simulink model "simRouteA_v4_11"  (R2015a)
settings: Solver=FixedStepDiscrete  StartTime=0.0  StopTime=36000  FixedStep=1  RelTol=1e-3
PreLoadFcn:
  | loadTimetable
StopFcn:
  | postProcess
undefined symbols (not defined in the file or in its folder): setBus1IntergenTime, setBus2IntergenTime, setBus3IntergenTime, setBus4IntergenTime
(part 6 of 7)

== system simRouteA_v4_11/chkSchedTimeNormalBusAtCP3/Subsystem2 ==
  ID : Inport
  tTable : Inport  Port=2
  Constant12 : Constant  Value=10000
  Constant13 : Constant
  Direct Lookup Table (n-D)1 : LookupNDDirect  TableIsInput=on
  Divide1 : Product  Inputs=/*
  Math Function1 : Math  Operator=mod  SaturateOnIntegerOverflow=on
  Rounding : Rounding  Operator=round
  Rounding1 : Rounding  Operator=round
  Subtract1 : Sum  Inputs=-+
  schedTime : Outport
  wires:
  Rounding1/1 -> Direct Lookup Table (n-D)1/1
  Constant12/1 -> Math Function1/2, Divide1/1
  Constant13/1 -> Subtract1/1
  Divide1/1 -> Rounding/1
  Subtract1/1 -> Direct Lookup Table (n-D)1/2
  Direct Lookup Table (n-D)1/1 -> schedTime/1
  tTable/1 -> Direct Lookup Table (n-D)1/3
  Math Function1/1 -> Rounding1/1
  Rounding/1 -> Subtract1/2
  ID/1 -> Divide1/2, Math Function1/1

== system simRouteA_v4_11/chkSchedTimeNormalBusAtCP3/While Iterator Subsystem ==
  crnBusID : Inport
  timetableAtStart : Inport  Port=2
  crnTimeAtCP : Inport  Port=3
  IC : Inport  Port=4
  Add1 : Sum
  Constant2 : Constant  Value=10000
  Constant4 : Constant
  Direct Lookup Table (n-D)2 : LookupNDDirect  TableIsInput=on
  Divide2 : Product  Inputs=/*
  Math Function1 : Math  Operator=mod  SaturateOnIntegerOverflow=on
  Memory : Memory
  Relational Operator : RelationalOperator  Operator=<=  OutDataTypeStr=boolean
  Rounding2 : Rounding  Operator=round
  Rounding3 : Rounding  Operator=round
  Subtract2 : Sum  Inputs=-+
  Sum : Sum  Inputs=|++
  While Iterator : WhileIterator  ShowIterationPort=on
  nxtDepTimeAtStart : Outport
  nxtBusID : Outport  Port=2
  wires:
  IC/1 -> While Iterator/2
  While Iterator/1 -> Sum/1
  Memory/1 -> Sum/2
  Sum/1 -> Add1/2, Memory/1
  crnBusID/1 -> Add1/1
  Rounding2/1 -> Direct Lookup Table (n-D)2/1
  Divide2/1 -> Rounding3/1
  Add1/1 -> Divide2/2, nxtBusID/1, Math Function1/1
  Math Function1/1 -> Rounding2/1
  Constant2/1 -> Divide2/1, Math Function1/2
  timetableAtStart/1 -> Direct Lookup Table (n-D)2/3
  Rounding3/1 -> Subtract2/2
  Constant4/1 -> Subtract2/1
  Subtract2/1 -> Direct Lookup Table (n-D)2/2
  Direct Lookup Table (n-D)2/1 -> Relational Operator/1, nxtDepTimeAtStart/1
  crnTimeAtCP/1 -> Relational Operator/2
  Relational Operator/1 -> While Iterator/1

== system simRouteA_v4_11/chkSchedTimeNormalBusAtCP4/Subsystem2 ==
  ID : Inport
  tTable : Inport  Port=2
  Constant12 : Constant  Value=10000
  Constant13 : Constant
  Direct Lookup Table (n-D)1 : LookupNDDirect  TableIsInput=on
  Divide1 : Product  Inputs=/*
  Math Function1 : Math  Operator=mod  SaturateOnIntegerOverflow=on
  Rounding : Rounding  Operator=round
  Rounding1 : Rounding  Operator=round
  Subtract1 : Sum  Inputs=-+
  schedTime : Outport
  wires:
  Rounding1/1 -> Direct Lookup Table (n-D)1/1
  Constant12/1 -> Math Function1/2, Divide1/1
  Constant13/1 -> Subtract1/1
  Divide1/1 -> Rounding/1
  Subtract1/1 -> Direct Lookup Table (n-D)1/2
  Direct Lookup Table (n-D)1/1 -> schedTime/1
  tTable/1 -> Direct Lookup Table (n-D)1/3
  Math Function1/1 -> Rounding1/1
  Rounding/1 -> Subtract1/2
  ID/1 -> Divide1/2, Math Function1/1

== system simRouteA_v4_11/chkSchedTimeNormalBusAtCP4/While Iterator Subsystem ==
  crnBusID : Inport
  timetableAtStart : Inport  Port=2
  crnTimeAtCP : Inport  Port=3
  IC : Inport  Port=4
  Add1 : Sum
  Constant2 : Constant  Value=10000
  Constant4 : Constant
  Direct Lookup Table (n-D)2 : LookupNDDirect  TableIsInput=on
  Divide2 : Product  Inputs=/*
  Math Function1 : Math  Operator=mod  SaturateOnIntegerOverflow=on
  Memory : Memory
  Relational Operator : RelationalOperator  Operator=<=  OutDataTypeStr=boolean
  Rounding2 : Rounding  Operator=round
  Rounding3 : Rounding  Operator=round
  Subtract2 : Sum  Inputs=-+
  Sum : Sum  Inputs=|++
  While Iterator : WhileIterator  ShowIterationPort=on
  nxtDepTimeAtStart : Outport
  nxtBusID : Outport  Port=2
  wires:
  IC/1 -> While Iterator/2
  While Iterator/1 -> Sum/1
  Memory/1 -> Sum/2
  Sum/1 -> Add1/2, Memory/1
  crnBusID/1 -> Add1/1
  Rounding2/1 -> Direct Lookup Table (n-D)2/1
  Divide2/1 -> Rounding3/1
  Add1/1 -> Divide2/2, nxtBusID/1, Math Function1/1
  Math Function1/1 -> Rounding2/1
  Constant2/1 -> Divide2/1, Math Function1/2
  timetableAtStart/1 -> Direct Lookup Table (n-D)2/3
  Rounding3/1 -> Subtract2/2
  Constant4/1 -> Subtract2/1
  Subtract2/1 -> Direct Lookup Table (n-D)2/2
  Direct Lookup Table (n-D)2/1 -> Relational Operator/1, nxtDepTimeAtStart/1
  crnTimeAtCP/1 -> Relational Operator/2
  Relational Operator/1 -> While Iterator/1

== system simRouteA_v4_11/holdBusAtCP2/While Iterator Subsystem ==
  crnBusID : Inport
  timetableAtStart : Inport  Port=2
  crnTimeAtCP : Inport  Port=3
  IC : Inport  Port=4
  Add1 : Sum
  Constant2 : Constant  Value=10000
  Constant4 : Constant
  Direct Lookup Table (n-D)2 : LookupNDDirect  TableIsInput=on
  Divide2 : Product  Inputs=/*
  Math Function1 : Math  Operator=mod  SaturateOnIntegerOverflow=on
  Memory : Memory
  Relational Operator : RelationalOperator  Operator=<=  OutDataTypeStr=boolean
  Rounding2 : Rounding  Operator=round
  Rounding3 : Rounding  Operator=round
  Subtract2 : Sum  Inputs=-+
  Sum : Sum  Inputs=|++
  While Iterator : WhileIterator  ShowIterationPort=on
  nxtDepTimeAtStart : Outport
  nxtBusID : Outport  Port=2
  wires:
  IC/1 -> While Iterator/2
  While Iterator/1 -> Sum/1
  Memory/1 -> Sum/2
  Sum/1 -> Add1/2, Memory/1
  crnBusID/1 -> Add1/1
  Rounding2/1 -> Direct Lookup Table (n-D)2/1
  Divide2/1 -> Rounding3/1
  Add1/1 -> Divide2/2, nxtBusID/1, Math Function1/1
  Math Function1/1 -> Rounding2/1
  Constant2/1 -> Divide2/1, Math Function1/2
  timetableAtStart/1 -> Direct Lookup Table (n-D)2/3
  Rounding3/1 -> Subtract2/2
  Constant4/1 -> Subtract2/1
  Subtract2/1 -> Direct Lookup Table (n-D)2/2
  Direct Lookup Table (n-D)2/1 -> Relational Operator/1, nxtDepTimeAtStart/1
  crnTimeAtCP/1 -> Relational Operator/2
  Relational Operator/1 -> While Iterator/1

== system simRouteA_v4_11/holdBusAtCP2/calculateHoldTimeAtCP ==
  crnSchedAtCP : Inport
  time : Inport  Port=2
  Constant2 : Constant  Value=0
  MinMax : MinMax  Function=max  Inputs=2
  Subtract1 : Sum  Inputs=+-
  tHoldCrnBus : Outport
  wires:
  Subtract1/1 -> MinMax/1
  MinMax/1 -> tHoldCrnBus/1
  Constant2/1 -> MinMax/2
  time/1 -> Subtract1/2
  crnSchedAtCP/1 -> Subtract1/1

== system simRouteA_v4_11/holdBusAtCP3/While Iterator Subsystem ==
  crnBusID : Inport
  timetableAtStart : Inport  Port=2
  crnTimeAtCP : Inport  Port=3
  IC : Inport  Port=4
  Add1 : Sum
  Constant2 : Constant  Value=10000
  Constant4 : Constant
  Direct Lookup Table (n-D)2 : LookupNDDirect  TableIsInput=on
  Divide2 : Product  Inputs=/*
  Math Function1 : Math  Operator=mod  SaturateOnIntegerOverflow=on
  Memory : Memory
  Relational Operator : RelationalOperator  Operator=<=  OutDataTypeStr=boolean
  Rounding2 : Rounding  Operator=round
  Rounding3 : Rounding  Operator=round
  Subtract2 : Sum  Inputs=-+
  Sum : Sum  Inputs=|++
  While Iterator : WhileIterator  ShowIterationPort=on
  nxtDepTimeAtStart : Outport
  nxtBusID : Outport  Port=2
  wires:
  IC/1 -> While Iterator/2
  While Iterator/1 -> Sum/1
  Memory/1 -> Sum/2
  Sum/1 -> Add1/2, Memory/1
  crnBusID/1 -> Add1/1
  Rounding2/1 -> Direct Lookup Table (n-D)2/1
  Divide2/1 -> Rounding3/1
  Add1/1 -> Divide2/2, nxtBusID/1, Math Function1/1
  Math Function1/1 -> Rounding2/1
  Constant2/1 -> Divide2/1, Math Function1/2
  timetableAtStart/1 -> Direct Lookup Table (n-D)2/3
  Rounding3/1 -> Subtract2/2
  Constant4/1 -> Subtract2/1
  Subtract2/1 -> Direct Lookup Table (n-D)2/2
  Direct Lookup Table (n-D)2/1 -> Relational Operator/1, nxtDepTimeAtStart/1
  crnTimeAtCP/1 -> Relational Operator/2
  Relational Operator/1 -> While Iterator/1

== system simRouteA_v4_11/holdBusAtCP3/calculateHoldTimeAtCP ==
  crnSchedAtCP : Inport
  time : Inport  Port=2
  Constant2 : Constant  Value=0
  MinMax : MinMax  Function=max  Inputs=2
  Subtract1 : Sum  Inputs=+-
  tHoldCrnBus : Outport
  wires:
  Subtract1/1 -> MinMax/1
  MinMax/1 -> tHoldCrnBus/1
  Constant2/1 -> MinMax/2
  time/1 -> Subtract1/2
  crnSchedAtCP/1 -> Subtract1/1

== system simRouteA_v4_11/holdBusAtCP4/While Iterator Subsystem ==
  crnBusID : Inport
  timetableAtStart : Inport  Port=2
  crnTimeAtCP : Inport  Port=3
  IC : Inport  Port=4
  Add1 : Sum
  Constant2 : Constant  Value=10000
  Constant4 : Constant
  Direct Lookup Table (n-D)2 : LookupNDDirect  TableIsInput=on
  Divide2 : Product  Inputs=/*
  Math Function1 : Math  Operator=mod  SaturateOnIntegerOverflow=on
  Memory : Memory
  Relational Operator : RelationalOperator  Operator=<=  OutDataTypeStr=boolean
  Rounding2 : Rounding  Operator=round
  Rounding3 : Rounding  Operator=round
  Subtract2 : Sum  Inputs=-+
  Sum : Sum  Inputs=|++
  While Iterator : WhileIterator  ShowIterationPort=on
  nxtDepTimeAtStart : Outport
  nxtBusID : Outport  Port=2
  wires:
  IC/1 -> While Iterator/2
  While Iterator/1 -> Sum/1
  Memory/1 -> Sum/2
  Sum/1 -> Add1/2, Memory/1
  crnBusID/1 -> Add1/1
  Rounding2/1 -> Direct Lookup Table (n-D)2/1
  Divide2/1 -> Rounding3/1
  Add1/1 -> Divide2/2, nxtBusID/1, Math Function1/1
  Math Function1/1 -> Rounding2/1
  Constant2/1 -> Divide2/1, Math Function1/2
  timetableAtStart/1 -> Direct Lookup Table (n-D)2/3
  Rounding3/1 -> Subtract2/2
  Constant4/1 -> Subtract2/1
  Subtract2/1 -> Direct Lookup Table (n-D)2/2
  Direct Lookup Table (n-D)2/1 -> Relational Operator/1, nxtDepTimeAtStart/1
  crnTimeAtCP/1 -> Relational Operator/2
  Relational Operator/1 -> While Iterator/1

== system simRouteA_v4_11/holdBusAtCP4/calculateHoldTimeAtCP ==
  crnSchedAtCP : Inport
  time : Inport  Port=2
  Constant2 : Constant  Value=0
  MinMax : MinMax  Function=max  Inputs=2
  Subtract1 : Sum  Inputs=+-
  tHoldCrnBus : Outport
  wires:
  Subtract1/1 -> MinMax/1
  MinMax/1 -> tHoldCrnBus/1
  Constant2/1 -> MinMax/2
  time/1 -> Subtract1/2
  crnSchedAtCP/1 -> Subtract1/1

== system simRouteA_v4_11/inTransitLinkL1/Subsystem2 ==
  tTrav : Inport
  tDep : Inport  Port=2
  Add1 : Sum
  Add2 : Sum
  Subtract : Sum  Inputs=+-
  Subtract1 : Sum  Inputs=+-
  Switch : Switch  Criteria=u2 > Threshold
  Unit Delay : UnitDelay  SampleTime=-1
  headWay : Constant  Value=3
  tTravNew : Outport
  wires:
  Subtract/1 -> Switch/2
  Switch/1 -> Subtract1/1, Unit Delay/1
  headWay/1 -> Add2/1
  tDep/1 -> Subtract1/2, Add1/2
  Add2/1 -> Switch/3
  tTrav/1 -> Add1/1
  Subtract1/1 -> tTravNew/1
  Add1/1 -> Switch/1, Subtract/1
  Unit Delay/1 -> Add2/2, Subtract/2

== system simRouteA_v4_11/inTransitLinkL10/Subsystem2 ==
  tTrav : Inport
  tDep : Inport  Port=2
  Add1 : Sum
  Add2 : Sum
  Subtract : Sum  Inputs=+-
  Subtract1 : Sum  Inputs=+-
  Switch : Switch  Criteria=u2 > Threshold
  Unit Delay : UnitDelay  SampleTime=-1
  headWay : Constant  Value=3
  tTravNew : Outport
  wires:
  Subtract/1 -> Switch/2
  Switch/1 -> Subtract1/1, Unit Delay/1
  headWay/1 -> Add2/1
  tDep/1 -> Subtract1/2, Add1/2
  Add2/1 -> Switch/3
  tTrav/1 -> Add1/1
  Subtract1/1 -> tTravNew/1
  Add1/1 -> Switch/1, Subtract/1
  Unit Delay/1 -> Add2/2, Subtract/2

== system simRouteA_v4_11/inTransitLinkL11/Subsystem2 ==
  tTrav : Inport
  tDep : Inport  Port=2
  Add1 : Sum
  Add2 : Sum
  Subtract : Sum  Inputs=+-
  Subtract1 : Sum  Inputs=+-
  Switch : Switch  Criteria=u2 > Threshold
  Unit Delay : UnitDelay  SampleTime=-1
  headWay : Constant  Value=3
  tTravNew : Outport
  wires:
  Subtract/1 -> Switch/2
  Switch/1 -> Subtract1/1, Unit Delay/1
  headWay/1 -> Add2/1
  tDep/1 -> Subtract1/2, Add1/2
  Add2/1 -> Switch/3
  tTrav/1 -> Add1/1
  Subtract1/1 -> tTravNew/1
  Add1/1 -> Switch/1, Subtract/1
  Unit Delay/1 -> Add2/2, Subtract/2

== system simRouteA_v4_11/inTransitLinkL12/Subsystem2 ==
  tTrav : Inport
  tDep : Inport  Port=2
  Add1 : Sum
  Add2 : Sum
  Subtract : Sum  Inputs=+-
  Subtract1 : Sum  Inputs=+-
  Switch : Switch  Criteria=u2 > Threshold
  Unit Delay : UnitDelay  SampleTime=-1
  headWay : Constant  Value=3
  tTravNew : Outport
  wires:
  Subtract/1 -> Switch/2
  Switch/1 -> Subtract1/1, Unit Delay/1
  headWay/1 -> Add2/1
  tDep/1 -> Subtract1/2, Add1/2
  Add2/1 -> Switch/3
  tTrav/1 -> Add1/1
  Subtract1/1 -> tTravNew/1
  Add1/1 -> Switch/1, Subtract/1
  Unit Delay/1 -> Add2/2, Subtract/2

== system simRouteA_v4_11/inTransitLinkL13/Subsystem2 ==
  tTrav : Inport
  tDep : Inport  Port=2
  Add1 : Sum
  Add2 : Sum
  Subtract : Sum  Inputs=+-
  Subtract1 : Sum  Inputs=+-
  Switch : Switch  Criteria=u2 > Threshold
  Unit Delay : UnitDelay  SampleTime=-1
  headWay : Constant  Value=3
  tTravNew : Outport
  wires:
  Subtract/1 -> Switch/2
  Switch/1 -> Subtract1/1, Unit Delay/1
  headWay/1 -> Add2/1
  tDep/1 -> Subtract1/2, Add1/2
  Add2/1 -> Switch/3
  tTrav/1 -> Add1/1
  Subtract1/1 -> tTravNew/1
  Add1/1 -> Switch/1, Subtract/1
  Unit Delay/1 -> Add2/2, Subtract/2

== system simRouteA_v4_11/inTransitLinkL14/Subsystem2 ==
  tTrav : Inport
  tDep : Inport  Port=2
  Add1 : Sum
  Add2 : Sum
  Subtract : Sum  Inputs=+-
  Subtract1 : Sum  Inputs=+-
  Switch : Switch  Criteria=u2 > Threshold
  Unit Delay : UnitDelay  SampleTime=-1
  headWay : Constant  Value=3
  tTravNew : Outport
  wires:
  Subtract/1 -> Switch/2
  Switch/1 -> Subtract1/1, Unit Delay/1
  headWay/1 -> Add2/1
  tDep/1 -> Subtract1/2, Add1/2
  Add2/1 -> Switch/3
  tTrav/1 -> Add1/1
  Subtract1/1 -> tTravNew/1
  Add1/1 -> Switch/1, Subtract/1
  Unit Delay/1 -> Add2/2, Subtract/2

== system simRouteA_v4_11/inTransitLinkL15/Subsystem2 ==
  tTrav : Inport
  tDep : Inport  Port=2
  Add1 : Sum
  Add2 : Sum
  Subtract : Sum  Inputs=+-
  Subtract1 : Sum  Inputs=+-
  Switch : Switch  Criteria=u2 > Threshold
  Unit Delay : UnitDelay  SampleTime=-1
  headWay : Constant  Value=3
  tTravNew : Outport
  wires:
  Subtract/1 -> Switch/2
  Switch/1 -> Subtract1/1, Unit Delay/1
  headWay/1 -> Add2/1
  tDep/1 -> Subtract1/2, Add1/2
  Add2/1 -> Switch/3
  tTrav/1 -> Add1/1
  Subtract1/1 -> tTravNew/1
  Add1/1 -> Switch/1, Subtract/1
  Unit Delay/1 -> Add2/2, Subtract/2

== system simRouteA_v4_11/inTransitLinkL16/Subsystem2 ==
  tTrav : Inport
  tDep : Inport  Port=2
  Add1 : Sum
  Add2 : Sum
  Subtract : Sum  Inputs=+-
  Subtract1 : Sum  Inputs=+-
  Switch : Switch  Criteria=u2 > Threshold
  Unit Delay : UnitDelay  SampleTime=-1
  headWay : Constant  Value=3
  tTravNew : Outport
  wires:
  Subtract/1 -> Switch/2
  Switch/1 -> Subtract1/1, Unit Delay/1
  headWay/1 -> Add2/1
  tDep/1 -> Subtract1/2, Add1/2
  Add2/1 -> Switch/3
  tTrav/1 -> Add1/1
  Subtract1/1 -> tTravNew/1
  Add1/1 -> Switch/1, Subtract/1
  Unit Delay/1 -> Add2/2, Subtract/2

== system simRouteA_v4_11/inTransitLinkL17/Subsystem2 ==
  tTrav : Inport
  tDep : Inport  Port=2
  Add1 : Sum
  Add2 : Sum
  Subtract : Sum  Inputs=+-
  Subtract1 : Sum  Inputs=+-
  Switch : Switch  Criteria=u2 > Threshold
  Unit Delay : UnitDelay  SampleTime=-1
  headWay : Constant  Value=3
  tTravNew : Outport
  wires:
  Subtract/1 -> Switch/2
  Switch/1 -> Subtract1/1, Unit Delay/1
  headWay/1 -> Add2/1
  tDep/1 -> Subtract1/2, Add1/2
  Add2/1 -> Switch/3
  tTrav/1 -> Add1/1
  Subtract1/1 -> tTravNew/1
  Add1/1 -> Switch/1, Subtract/1
  Unit Delay/1 -> Add2/2, Subtract/2

== system simRouteA_v4_11/inTransitLinkL18/Subsystem2 ==
  tTrav : Inport
  tDep : Inport  Port=2
  Add1 : Sum
  Add2 : Sum
  Subtract : Sum  Inputs=+-
  Subtract1 : Sum  Inputs=+-
  Switch : Switch  Criteria=u2 > Threshold
  Unit Delay : UnitDelay  SampleTime=-1
  headWay : Constant  Value=3
  tTravNew : Outport
  wires:
  Subtract/1 -> Switch/2
  Switch/1 -> Subtract1/1, Unit Delay/1
  headWay/1 -> Add2/1
  tDep/1 -> Subtract1/2, Add1/2
  Add2/1 -> Switch/3
  tTrav/1 -> Add1/1
  Subtract1/1 -> tTravNew/1
  Add1/1 -> Switch/1, Subtract/1
  Unit Delay/1 -> Add2/2, Subtract/2

== system simRouteA_v4_11/inTransitLinkL2/Subsystem2 ==
  tTrav : Inport
  tDep : Inport  Port=2
  Add1 : Sum
  Add2 : Sum
  Subtract : Sum  Inputs=+-
  Subtract1 : Sum  Inputs=+-
  Switch : Switch  Criteria=u2 > Threshold
  Unit Delay : UnitDelay  SampleTime=-1
  headWay : Constant  Value=3
  tTravNew : Outport
  wires:
  Subtract/1 -> Switch/2
  Switch/1 -> Subtract1/1, Unit Delay/1
  headWay/1 -> Add2/1
  tDep/1 -> Subtract1/2, Add1/2
  Add2/1 -> Switch/3
  tTrav/1 -> Add1/1
  Subtract1/1 -> tTravNew/1
  Add1/1 -> Switch/1, Subtract/1
  Unit Delay/1 -> Add2/2, Subtract/2

== system simRouteA_v4_11/inTransitLinkL3/Subsystem2 ==
  tTrav : Inport
  tDep : Inport  Port=2
  Add1 : Sum
  Add2 : Sum
  Subtract : Sum  Inputs=+-
  Subtract1 : Sum  Inputs=+-
  Switch : Switch  Criteria=u2 > Threshold
  Unit Delay : UnitDelay  SampleTime=-1
  headWay : Constant  Value=3
  tTravNew : Outport
  wires:
  Subtract/1 -> Switch/2
  Switch/1 -> Subtract1/1, Unit Delay/1
  headWay/1 -> Add2/1
  tDep/1 -> Subtract1/2, Add1/2
  Add2/1 -> Switch/3
  tTrav/1 -> Add1/1
  Subtract1/1 -> tTravNew/1
  Add1/1 -> Switch/1, Subtract/1
  Unit Delay/1 -> Add2/2, Subtract/2

== system simRouteA_v4_11/inTransitLinkL4/Subsystem2 ==
  tTrav : Inport
  tDep : Inport  Port=2
  Add1 : Sum
  Add2 : Sum
  Subtract : Sum  Inputs=+-
  Subtract1 : Sum  Inputs=+-
  Switch : Switch  Criteria=u2 > Threshold
  Unit Delay : UnitDelay  SampleTime=-1
  headWay : Constant  Value=3
  tTravNew : Outport
  wires:
  Subtract/1 -> Switch/2
  Switch/1 -> Subtract1/1, Unit Delay/1
  headWay/1 -> Add2/1
  tDep/1 -> Subtract1/2, Add1/2
  Add2/1 -> Switch/3
  tTrav/1 -> Add1/1
  Subtract1/1 -> tTravNew/1
  Add1/1 -> Switch/1, Subtract/1
  Unit Delay/1 -> Add2/2, Subtract/2

== system simRouteA_v4_11/inTransitLinkL5/Subsystem2 ==
  tTrav : Inport
  tDep : Inport  Port=2
  Add1 : Sum
  Add2 : Sum
  Subtract : Sum  Inputs=+-
  Subtract1 : Sum  Inputs=+-
  Switch : Switch  Criteria=u2 > Threshold
  Unit Delay : UnitDelay  SampleTime=-1
  headWay : Constant  Value=3
  tTravNew : Outport
  wires:
  Subtract/1 -> Switch/2
  Switch/1 -> Subtract1/1, Unit Delay/1
  headWay/1 -> Add2/1
  tDep/1 -> Subtract1/2, Add1/2
  Add2/1 -> Switch/3
  tTrav/1 -> Add1/1
  Subtract1/1 -> tTravNew/1
  Add1/1 -> Switch/1, Subtract/1
  Unit Delay/1 -> Add2/2, Subtract/2

== system simRouteA_v4_11/inTransitLinkL6/Subsystem2 ==
  tTrav : Inport
  tDep : Inport  Port=2
  Add1 : Sum
  Add2 : Sum
  Subtract : Sum  Inputs=+-
  Subtract1 : Sum  Inputs=+-
  Switch : Switch  Criteria=u2 > Threshold
  Unit Delay : UnitDelay  SampleTime=-1
  headWay : Constant  Value=3
  tTravNew : Outport
  wires:
  Subtract/1 -> Switch/2
  Switch/1 -> Subtract1/1, Unit Delay/1
  headWay/1 -> Add2/1
  tDep/1 -> Subtract1/2, Add1/2
  Add2/1 -> Switch/3
  tTrav/1 -> Add1/1
  Subtract1/1 -> tTravNew/1
  Add1/1 -> Switch/1, Subtract/1
  Unit Delay/1 -> Add2/2, Subtract/2

== system simRouteA_v4_11/inTransitLinkL7/Subsystem2 ==
  tTrav : Inport
  tDep : Inport  Port=2
  Add1 : Sum
  Add2 : Sum
  Subtract : Sum  Inputs=+-
  Subtract1 : Sum  Inputs=+-
  Switch : Switch  Criteria=u2 > Threshold
  Unit Delay : UnitDelay  SampleTime=-1
  headWay : Constant  Value=3
  tTravNew : Outport
  wires:
  Subtract/1 -> Switch/2
  Switch/1 -> Subtract1/1, Unit Delay/1
  headWay/1 -> Add2/1
  tDep/1 -> Subtract1/2, Add1/2
  Add2/1 -> Switch/3
  tTrav/1 -> Add1/1
  Subtract1/1 -> tTravNew/1
  Add1/1 -> Switch/1, Subtract/1
  Unit Delay/1 -> Add2/2, Subtract/2

== system simRouteA_v4_11/inTransitLinkL8/Subsystem2 ==
  tTrav : Inport
  tDep : Inport  Port=2
  Add1 : Sum
  Add2 : Sum
  Subtract : Sum  Inputs=+-
  Subtract1 : Sum  Inputs=+-
  Switch : Switch  Criteria=u2 > Threshold
  Unit Delay : UnitDelay  SampleTime=-1
  headWay : Constant  Value=3
  tTravNew : Outport
  wires:
  Subtract/1 -> Switch/2
  Switch/1 -> Subtract1/1, Unit Delay/1
  headWay/1 -> Add2/1
  tDep/1 -> Subtract1/2, Add1/2
  Add2/1 -> Switch/3
  tTrav/1 -> Add1/1
  Subtract1/1 -> tTravNew/1
  Add1/1 -> Switch/1, Subtract/1
  Unit Delay/1 -> Add2/2, Subtract/2

== system simRouteA_v4_11/inTransitLinkL9/Subsystem2 ==
  tTrav : Inport
  tDep : Inport  Port=2
  Add1 : Sum
  Add2 : Sum
  Subtract : Sum  Inputs=+-
  Subtract1 : Sum  Inputs=+-
  Switch : Switch  Criteria=u2 > Threshold
  Unit Delay : UnitDelay  SampleTime=-1
  headWay : Constant  Value=3
  tTravNew : Outport
  wires:
  Subtract/1 -> Switch/2
  Switch/1 -> Subtract1/1, Unit Delay/1
  headWay/1 -> Add2/1
  tDep/1 -> Subtract1/2, Add1/2
  Add2/1 -> Switch/3
  tTrav/1 -> Add1/1
  Subtract1/1 -> tTravNew/1
  Add1/1 -> Switch/1, Subtract/1
  Unit Delay/1 -> Add2/2, Subtract/2

== system simRouteA_v4_11/atStopS1/busDwellThisStop/Subsystem2 ==
  dwellTime : Inport
  tStartSrvPax : Inport  Port=2
  Add1 : Sum
  Add2 : Sum
  Subtract : Sum  Inputs=+-
  Subtract1 : Sum  Inputs=+-
  Switch : Switch  Criteria=u2 > Threshold
  Unit Delay : UnitDelay  SampleTime=-1
  headWay : Constant  Value=3
  dwellTimeNew : Outport
  wires:
  Subtract/1 -> Switch/2
  Switch/1 -> Subtract1/1, Unit Delay/1
  headWay/1 -> Add2/1
  tStartSrvPax/1 -> Subtract1/2, Add1/2
  Add2/1 -> Switch/3
  dwellTime/1 -> Add1/1
  Subtract1/1 -> dwellTimeNew/1
  Add1/1 -> Switch/1, Subtract/1
  Unit Delay/1 -> Add2/2, Subtract/2

== system simRouteA_v4_11/atStopS1/calcPaxActivThisStop/Atomic Subsystem ==
  maxCap : Inport
  vacancy : Inport  Port=2
  paxAlight : Inport  Port=3
  paxArr : Inport  Port=4
  sec2Brd : Inport  Port=5
  Add : Sum
  Add1 : Sum
  Add2 : Sum
  Initial Value : InitialValue  Commented=on  InitialValue=0
  Min1 : MinMax  Inputs=2
  Min2 : MinMax  Inputs=2
  Product : Product
  Signal Latch : SignalLatch  Commented=on  MemoryWriteEdgeOption=Either  MemoryReadEdgeOption=Either  SpecifyReadEventPriority=on
      settings: InputPortMap=u0,u1,u2  OutputPortMap=o2
  Subtract : Sum  Inputs=+-
  Subtract1 : Sum  Inputs=-+
  Subtract2 : Sum  Inputs=+-
  Unit Delay : UnitDelay  SampleTime=-1
  newVacancy : Outport
  paxBoard : Outport  Port=2
  paxRemain : Outport  Port=3
  paxWait : Outport  Port=4
  dwellTime : Outport  Port=5
  corrPaxAlight : Outport  Port=6
  wires:
  Add/1 -> Min1/1, Subtract/1
  Min1/1 -> Subtract1/1, Subtract/2, Add2/1, paxBoard/1
  paxArr/1 -> Add1/1
  Add1/1 -> paxWait/1, Subtract1/2, Min1/2
  Subtract1/1 -> Unit Delay/1, paxRemain/1
  Unit Delay/1 -> Add1/2
  vacancy/1 -> Subtract2/2, Add/1
  maxCap/1 -> Subtract2/1
  Subtract/1 -> newVacancy/1
  Add2/1 -> Product/1
  sec2Brd/1 -> Product/2
  Product/1 -> dwellTime/1
  Subtract2/1 -> Min2/1
  Min2/1 -> corrPaxAlight/1, Add2/2, Add/2
  paxAlight/1 -> Min2/2

== system simRouteA_v4_11/atStopS1/calcPaxActivThisStop/calcPaxAlightS1 ==
  integrPax : Inport
  Subtract : Sum  Inputs=+-
  Unit Delay : UnitDelay  SampleTime=-1
  truPax : Outport
  intgPax : Outport  Port=2
  wires:
  integrPax/1 -> Unit Delay/1, intgPax/1, Subtract/1
  Subtract/1 -> truPax/1
  Unit Delay/1 -> Subtract/2

== system simRouteA_v4_11/atStopS1/calcPaxActivThisStop/calcPaxArrS1 ==
  integrPax : Inport
  Subtract : Sum  Inputs=+-
  Unit Delay : UnitDelay  SampleTime=-1
  truPax : Outport
  intgPax : Outport  Port=2
  wires:
  integrPax/1 -> Unit Delay/1, intgPax/1, Subtract/1
  Subtract/1 -> truPax/1
  Unit Delay/1 -> Subtract/2

== system simRouteA_v4_11/atStopS1/integrPaxAlightS1/Atomic Subsystem1 ==
  In1 : Inport
  Add : Sum
  Unit Delay : UnitDelay  SampleTime=-1
  Out1 : Outport
  wires:
  In1/1 -> Add/1
  Add/1 -> Out1/1, Unit Delay/1
  Unit Delay/1 -> Add/2

== system simRouteA_v4_11/atStopS1/integrPaxArrS1/Atomic Subsystem1 ==
  In1 : Inport
  Add : Sum
  Unit Delay : UnitDelay  SampleTime=-1
  Out1 : Outport
  wires:
  In1/1 -> Add/1
  Add/1 -> Out1/1, Unit Delay/1
  Unit Delay/1 -> Add/2

== system simRouteA_v4_11/atStopS10/busDwellThisStop/Subsystem2 ==
  dwellTime : Inport
  tStartSrvPax : Inport  Port=2
  Add1 : Sum
  Add2 : Sum
  Subtract : Sum  Inputs=+-
  Subtract1 : Sum  Inputs=+-
  Switch : Switch  Criteria=u2 > Threshold
  Unit Delay : UnitDelay  SampleTime=-1
  headWay : Constant  Value=3
  dwellTimeNew : Outport
  wires:
  Subtract/1 -> Switch/2
  Switch/1 -> Subtract1/1, Unit Delay/1
  headWay/1 -> Add2/1
  tStartSrvPax/1 -> Subtract1/2, Add1/2
  Add2/1 -> Switch/3
  dwellTime/1 -> Add1/1
  Subtract1/1 -> dwellTimeNew/1
  Add1/1 -> Switch/1, Subtract/1
  Unit Delay/1 -> Add2/2, Subtract/2

== system simRouteA_v4_11/atStopS10/calcPaxActivThisStop/Atomic Subsystem ==
  maxCap : Inport
  vacancy : Inport  Port=2
  paxAlight : Inport  Port=3
  paxArr : Inport  Port=4
  sec2Brd : Inport  Port=5
  Add : Sum
  Add1 : Sum
  Add2 : Sum
  Initial Value : InitialValue  Commented=on  InitialValue=0
  Min1 : MinMax  Inputs=2
  Min2 : MinMax  Inputs=2
  Product : Product
  Signal Latch : SignalLatch  Commented=on  MemoryWriteEdgeOption=Either  MemoryReadEdgeOption=Either  SpecifyReadEventPriority=on
      settings: InputPortMap=u0,u1,u2  OutputPortMap=o2
  Subtract : Sum  Inputs=+-
  Subtract1 : Sum  Inputs=-+
  Subtract2 : Sum  Inputs=+-
  Unit Delay : UnitDelay  SampleTime=-1
  newVacancy : Outport
  paxBoard : Outport  Port=2
  paxRemain : Outport  Port=3
  paxWait : Outport  Port=4
  dwellTime : Outport  Port=5
  corrPaxAlight : Outport  Port=6
  wires:
  Add/1 -> Min1/1, Subtract/1
  Min1/1 -> Subtract1/1, Subtract/2, Add2/1, paxBoard/1
  paxArr/1 -> Add1/1
  Add1/1 -> paxWait/1, Subtract1/2, Min1/2
  Subtract1/1 -> Unit Delay/1, paxRemain/1
  Unit Delay/1 -> Add1/2
  vacancy/1 -> Subtract2/2, Add/1
  maxCap/1 -> Subtract2/1
  Subtract/1 -> newVacancy/1
  Add2/1 -> Product/1
  sec2Brd/1 -> Product/2
  Product/1 -> dwellTime/1
  Subtract2/1 -> Min2/1
  Min2/1 -> corrPaxAlight/1, Add2/2, Add/2
  paxAlight/1 -> Min2/2

== system simRouteA_v4_11/atStopS10/calcPaxActivThisStop/calcPaxAlightS1 ==
  integrPax : Inport
  Subtract : Sum  Inputs=+-
  Unit Delay : UnitDelay  SampleTime=-1
  truPax : Outport
  intgPax : Outport  Port=2
  wires:
  integrPax/1 -> Unit Delay/1, intgPax/1, Subtract/1
  Subtract/1 -> truPax/1
  Unit Delay/1 -> Subtract/2

== system simRouteA_v4_11/atStopS10/calcPaxActivThisStop/calcPaxArrS1 ==
  integrPax : Inport
  Subtract : Sum  Inputs=+-
  Unit Delay : UnitDelay  SampleTime=-1
  truPax : Outport
  intgPax : Outport  Port=2
  wires:
  integrPax/1 -> Unit Delay/1, intgPax/1, Subtract/1
  Subtract/1 -> truPax/1
  Unit Delay/1 -> Subtract/2

== system simRouteA_v4_11/atStopS10/integrPaxAlightS1/Atomic Subsystem1 ==
  In1 : Inport
  Add : Sum
  Unit Delay : UnitDelay  SampleTime=-1
  Out1 : Outport
  wires:
  In1/1 -> Add/1
  Add/1 -> Out1/1, Unit Delay/1
  Unit Delay/1 -> Add/2

== system simRouteA_v4_11/atStopS10/integrPaxArrS1/Atomic Subsystem1 ==
  In1 : Inport
  Add : Sum
  Unit Delay : UnitDelay  SampleTime=-1
  Out1 : Outport
  wires:
  In1/1 -> Add/1
  Add/1 -> Out1/1, Unit Delay/1
  Unit Delay/1 -> Add/2

== system simRouteA_v4_11/atStopS11/busDwellThisStop/Subsystem2 ==
  dwellTime : Inport
  tStartSrvPax : Inport  Port=2
  Add1 : Sum
  Add2 : Sum
  Subtract : Sum  Inputs=+-
  Subtract1 : Sum  Inputs=+-
  Switch : Switch  Criteria=u2 > Threshold
  Unit Delay : UnitDelay  SampleTime=-1
  headWay : Constant  Value=3
  dwellTimeNew : Outport
  wires:
  Subtract/1 -> Switch/2
  Switch/1 -> Subtract1/1, Unit Delay/1
  headWay/1 -> Add2/1
  tStartSrvPax/1 -> Subtract1/2, Add1/2
  Add2/1 -> Switch/3
  dwellTime/1 -> Add1/1
  Subtract1/1 -> dwellTimeNew/1
  Add1/1 -> Switch/1, Subtract/1
  Unit Delay/1 -> Add2/2, Subtract/2

== system simRouteA_v4_11/atStopS11/calcPaxActivThisStop/Atomic Subsystem ==
  maxCap : Inport
  vacancy : Inport  Port=2
  paxAlight : Inport  Port=3
  paxArr : Inport  Port=4
  sec2Brd : Inport  Port=5
  Add : Sum
  Add1 : Sum
  Add2 : Sum
  Initial Value : InitialValue  Commented=on  InitialValue=0
  Min1 : MinMax  Inputs=2
  Min2 : MinMax  Inputs=2
  Product : Product
  Signal Latch : SignalLatch  Commented=on  MemoryWriteEdgeOption=Either  MemoryReadEdgeOption=Either  SpecifyReadEventPriority=on
      settings: InputPortMap=u0,u1,u2  OutputPortMap=o2
  Subtract : Sum  Inputs=+-
  Subtract1 : Sum  Inputs=-+
  Subtract2 : Sum  Inputs=+-
  Unit Delay : UnitDelay  SampleTime=-1
  newVacancy : Outport
  paxBoard : Outport  Port=2
  paxRemain : Outport  Port=3
  paxWait : Outport  Port=4
  dwellTime : Outport  Port=5
  corrPaxAlight : Outport  Port=6
  wires:
  Add/1 -> Min1/1, Subtract/1
  Min1/1 -> Subtract1/1, Subtract/2, Add2/1, paxBoard/1
  paxArr/1 -> Add1/1
  Add1/1 -> paxWait/1, Subtract1/2, Min1/2
  Subtract1/1 -> Unit Delay/1, paxRemain/1
  Unit Delay/1 -> Add1/2
  vacancy/1 -> Subtract2/2, Add/1
  maxCap/1 -> Subtract2/1
  Subtract/1 -> newVacancy/1
  Add2/1 -> Product/1
  sec2Brd/1 -> Product/2
  Product/1 -> dwellTime/1
  Subtract2/1 -> Min2/1
  Min2/1 -> corrPaxAlight/1, Add2/2, Add/2
  paxAlight/1 -> Min2/2

== system simRouteA_v4_11/atStopS11/calcPaxActivThisStop/calcPaxAlightS1 ==
  integrPax : Inport
  Subtract : Sum  Inputs=+-
  Unit Delay : UnitDelay  SampleTime=-1
  truPax : Outport
  intgPax : Outport  Port=2
  wires:
  integrPax/1 -> Unit Delay/1, intgPax/1, Subtract/1
  Subtract/1 -> truPax/1
  Unit Delay/1 -> Subtract/2

== system simRouteA_v4_11/atStopS11/calcPaxActivThisStop/calcPaxArrS1 ==
  integrPax : Inport
  Subtract : Sum  Inputs=+-
  Unit Delay : UnitDelay  SampleTime=-1
  truPax : Outport
  intgPax : Outport  Port=2
  wires:
  integrPax/1 -> Unit Delay/1, intgPax/1, Subtract/1
  Subtract/1 -> truPax/1
  Unit Delay/1 -> Subtract/2

== system simRouteA_v4_11/atStopS11/integrPaxAlightS1/Atomic Subsystem1 ==
  In1 : Inport
  Add : Sum
  Unit Delay : UnitDelay  SampleTime=-1
  Out1 : Outport
  wires:
  In1/1 -> Add/1
  Add/1 -> Out1/1, Unit Delay/1
  Unit Delay/1 -> Add/2

== system simRouteA_v4_11/atStopS11/integrPaxArrS1/Atomic Subsystem1 ==
  In1 : Inport
  Add : Sum
  Unit Delay : UnitDelay  SampleTime=-1
  Out1 : Outport
  wires:
  In1/1 -> Add/1
  Add/1 -> Out1/1, Unit Delay/1
  Unit Delay/1 -> Add/2

== system simRouteA_v4_11/atStopS12/busDwellThisStop/Subsystem2 ==
  dwellTime : Inport
  tStartSrvPax : Inport  Port=2
  Add1 : Sum
  Add2 : Sum
  Subtract : Sum  Inputs=+-
  Subtract1 : Sum  Inputs=+-
  Switch : Switch  Criteria=u2 > Threshold
  Unit Delay : UnitDelay  SampleTime=-1
  headWay : Constant  Value=3
  dwellTimeNew : Outport
  wires:
  Subtract/1 -> Switch/2
  Switch/1 -> Subtract1/1, Unit Delay/1
  headWay/1 -> Add2/1
  tStartSrvPax/1 -> Subtract1/2, Add1/2
  Add2/1 -> Switch/3
  dwellTime/1 -> Add1/1
  Subtract1/1 -> dwellTimeNew/1
  Add1/1 -> Switch/1, Subtract/1
  Unit Delay/1 -> Add2/2, Subtract/2

== system simRouteA_v4_11/atStopS12/calcPaxActivThisStop/Atomic Subsystem ==
  maxCap : Inport
  vacancy : Inport  Port=2
  paxAlight : Inport  Port=3
  paxArr : Inport  Port=4
  sec2Brd : Inport  Port=5
  Add : Sum
  Add1 : Sum
  Add2 : Sum
  Initial Value : InitialValue  Commented=on  InitialValue=0
  Min1 : MinMax  Inputs=2
  Min2 : MinMax  Inputs=2
  Product : Product
  Signal Latch : SignalLatch  Commented=on  MemoryWriteEdgeOption=Either  MemoryReadEdgeOption=Either  SpecifyReadEventPriority=on
      settings: InputPortMap=u0,u1,u2  OutputPortMap=o2
  Subtract : Sum  Inputs=+-
  Subtract1 : Sum  Inputs=-+
  Subtract2 : Sum  Inputs=+-
  Unit Delay : UnitDelay  SampleTime=-1
  newVacancy : Outport
  paxBoard : Outport  Port=2
  paxRemain : Outport  Port=3
  paxWait : Outport  Port=4
  dwellTime : Outport  Port=5
  corrPaxAlight : Outport  Port=6
  wires:
  Add/1 -> Min1/1, Subtract/1
  Min1/1 -> Subtract1/1, Subtract/2, Add2/1, paxBoard/1
  paxArr/1 -> Add1/1
  Add1/1 -> paxWait/1, Subtract1/2, Min1/2
  Subtract1/1 -> Unit Delay/1, paxRemain/1
  Unit Delay/1 -> Add1/2
  vacancy/1 -> Subtract2/2, Add/1
  maxCap/1 -> Subtract2/1
  Subtract/1 -> newVacancy/1
  Add2/1 -> Product/1
  sec2Brd/1 -> Product/2
  Product/1 -> dwellTime/1
  Subtract2/1 -> Min2/1
  Min2/1 -> corrPaxAlight/1, Add2/2, Add/2
  paxAlight/1 -> Min2/2

== system simRouteA_v4_11/atStopS12/calcPaxActivThisStop/calcPaxAlightS1 ==
  integrPax : Inport
  Subtract : Sum  Inputs=+-
  Unit Delay : UnitDelay  SampleTime=-1
  truPax : Outport
  intgPax : Outport  Port=2
  wires:
  integrPax/1 -> Unit Delay/1, intgPax/1, Subtract/1
  Subtract/1 -> truPax/1
  Unit Delay/1 -> Subtract/2

== system simRouteA_v4_11/atStopS12/calcPaxActivThisStop/calcPaxArrS1 ==
  integrPax : Inport
  Subtract : Sum  Inputs=+-
  Unit Delay : UnitDelay  SampleTime=-1
  truPax : Outport
  intgPax : Outport  Port=2
  wires:
  integrPax/1 -> Unit Delay/1, intgPax/1, Subtract/1
  Subtract/1 -> truPax/1
  Unit Delay/1 -> Subtract/2

== system simRouteA_v4_11/atStopS12/integrPaxAlightS1/Atomic Subsystem1 ==
  In1 : Inport
  Add : Sum
  Unit Delay : UnitDelay  SampleTime=-1
  Out1 : Outport
  wires:
  In1/1 -> Add/1
  Add/1 -> Out1/1, Unit Delay/1
  Unit Delay/1 -> Add/2

== system simRouteA_v4_11/atStopS12/integrPaxArrS1/Atomic Subsystem1 ==
  In1 : Inport
  Add : Sum
  Unit Delay : UnitDelay  SampleTime=-1
  Out1 : Outport
  wires:
  In1/1 -> Add/1
  Add/1 -> Out1/1, Unit Delay/1
  Unit Delay/1 -> Add/2

== system simRouteA_v4_11/atStopS13/busDwellThisStop/Subsystem2 ==
  dwellTime : Inport
  tStartSrvPax : Inport  Port=2
  Add1 : Sum
  Add2 : Sum
  Subtract : Sum  Inputs=+-
  Subtract1 : Sum  Inputs=+-
  Switch : Switch  Criteria=u2 > Threshold
  Unit Delay : UnitDelay  SampleTime=-1
  headWay : Constant  Value=3
  dwellTimeNew : Outport
  wires:
  Subtract/1 -> Switch/2
  Switch/1 -> Subtract1/1, Unit Delay/1
  headWay/1 -> Add2/1
  tStartSrvPax/1 -> Subtract1/2, Add1/2
  Add2/1 -> Switch/3
  dwellTime/1 -> Add1/1
  Subtract1/1 -> dwellTimeNew/1
  Add1/1 -> Switch/1, Subtract/1
  Unit Delay/1 -> Add2/2, Subtract/2

== system simRouteA_v4_11/atStopS13/calcPaxActivThisStop/Atomic Subsystem ==
  maxCap : Inport
  vacancy : Inport  Port=2
  paxAlight : Inport  Port=3
  paxArr : Inport  Port=4
  sec2Brd : Inport  Port=5
  Add : Sum
  Add1 : Sum
  Add2 : Sum
  Initial Value : InitialValue  Commented=on  InitialValue=0
  Min1 : MinMax  Inputs=2
  Min2 : MinMax  Inputs=2
  Product : Product
  Signal Latch : SignalLatch  Commented=on  MemoryWriteEdgeOption=Either  MemoryReadEdgeOption=Either  SpecifyReadEventPriority=on
      settings: InputPortMap=u0,u1,u2  OutputPortMap=o2
  Subtract : Sum  Inputs=+-
  Subtract1 : Sum  Inputs=-+
  Subtract2 : Sum  Inputs=+-
  Unit Delay : UnitDelay  SampleTime=-1
  newVacancy : Outport
  paxBoard : Outport  Port=2
  paxRemain : Outport  Port=3
  paxWait : Outport  Port=4
  dwellTime : Outport  Port=5
  corrPaxAlight : Outport  Port=6
  wires:
  Add/1 -> Min1/1, Subtract/1
  Min1/1 -> Subtract1/1, Subtract/2, Add2/1, paxBoard/1
  paxArr/1 -> Add1/1
  Add1/1 -> paxWait/1, Subtract1/2, Min1/2
  Subtract1/1 -> Unit Delay/1, paxRemain/1
  Unit Delay/1 -> Add1/2
  vacancy/1 -> Subtract2/2, Add/1
  maxCap/1 -> Subtract2/1
  Subtract/1 -> newVacancy/1
  Add2/1 -> Product/1
  sec2Brd/1 -> Product/2
  Product/1 -> dwellTime/1
  Subtract2/1 -> Min2/1
  Min2/1 -> corrPaxAlight/1, Add2/2, Add/2
  paxAlight/1 -> Min2/2

== system simRouteA_v4_11/atStopS13/calcPaxActivThisStop/calcPaxAlightS1 ==
  integrPax : Inport
  Subtract : Sum  Inputs=+-
  Unit Delay : UnitDelay  SampleTime=-1
  truPax : Outport
  intgPax : Outport  Port=2
  wires:
  integrPax/1 -> Unit Delay/1, intgPax/1, Subtract/1
  Subtract/1 -> truPax/1
  Unit Delay/1 -> Subtract/2

== system simRouteA_v4_11/atStopS13/calcPaxActivThisStop/calcPaxArrS1 ==
  integrPax : Inport
  Subtract : Sum  Inputs=+-
  Unit Delay : UnitDelay  SampleTime=-1
  truPax : Outport
  intgPax : Outport  Port=2
  wires:
  integrPax/1 -> Unit Delay/1, intgPax/1, Subtract/1
  Subtract/1 -> truPax/1
  Unit Delay/1 -> Subtract/2

== system simRouteA_v4_11/atStopS13/integrPaxAlightS1/Atomic Subsystem1 ==
  In1 : Inport
  Add : Sum
  Unit Delay : UnitDelay  SampleTime=-1
  Out1 : Outport
  wires:
  In1/1 -> Add/1
  Add/1 -> Out1/1, Unit Delay/1
  Unit Delay/1 -> Add/2

== system simRouteA_v4_11/atStopS13/integrPaxArrS1/Atomic Subsystem1 ==
  In1 : Inport
  Add : Sum
  Unit Delay : UnitDelay  SampleTime=-1
  Out1 : Outport
  wires:
  In1/1 -> Add/1
  Add/1 -> Out1/1, Unit Delay/1
  Unit Delay/1 -> Add/2

== system simRouteA_v4_11/atStopS14/busDwellThisStop/Subsystem2 ==
  dwellTime : Inport
  tStartSrvPax : Inport  Port=2
  Add1 : Sum
  Add2 : Sum
  Subtract : Sum  Inputs=+-
  Subtract1 : Sum  Inputs=+-
  Switch : Switch  Criteria=u2 > Threshold
  Unit Delay : UnitDelay  SampleTime=-1
  headWay : Constant  Value=3
  dwellTimeNew : Outport
  wires:
  Subtract/1 -> Switch/2
  Switch/1 -> Subtract1/1, Unit Delay/1
  headWay/1 -> Add2/1
  tStartSrvPax/1 -> Subtract1/2, Add1/2
  Add2/1 -> Switch/3
  dwellTime/1 -> Add1/1
  Subtract1/1 -> dwellTimeNew/1
  Add1/1 -> Switch/1, Subtract/1
  Unit Delay/1 -> Add2/2, Subtract/2

== system simRouteA_v4_11/atStopS14/calcPaxActivThisStop/Atomic Subsystem ==
  maxCap : Inport
  vacancy : Inport  Port=2
  paxAlight : Inport  Port=3
  paxArr : Inport  Port=4
  sec2Brd : Inport  Port=5
  Add : Sum
  Add1 : Sum
  Add2 : Sum
  Initial Value : InitialValue  Commented=on  InitialValue=0
  Min1 : MinMax  Inputs=2
  Min2 : MinMax  Inputs=2
  Product : Product
  Signal Latch : SignalLatch  Commented=on  MemoryWriteEdgeOption=Either  MemoryReadEdgeOption=Either  SpecifyReadEventPriority=on
      settings: InputPortMap=u0,u1,u2  OutputPortMap=o2
  Subtract : Sum  Inputs=+-
  Subtract1 : Sum  Inputs=-+
  Subtract2 : Sum  Inputs=+-
  Unit Delay : UnitDelay  SampleTime=-1
  newVacancy : Outport
  paxBoard : Outport  Port=2
  paxRemain : Outport  Port=3
  paxWait : Outport  Port=4
  dwellTime : Outport  Port=5
  corrPaxAlight : Outport  Port=6
  wires:
  Add/1 -> Min1/1, Subtract/1
  Min1/1 -> Subtract1/1, Subtract/2, Add2/1, paxBoard/1
  paxArr/1 -> Add1/1
  Add1/1 -> paxWait/1, Subtract1/2, Min1/2
  Subtract1/1 -> Unit Delay/1, paxRemain/1
  Unit Delay/1 -> Add1/2
  vacancy/1 -> Subtract2/2, Add/1
  maxCap/1 -> Subtract2/1
  Subtract/1 -> newVacancy/1
  Add2/1 -> Product/1
  sec2Brd/1 -> Product/2
  Product/1 -> dwellTime/1
  Subtract2/1 -> Min2/1
  Min2/1 -> corrPaxAlight/1, Add2/2, Add/2
  paxAlight/1 -> Min2/2

== system simRouteA_v4_11/atStopS14/calcPaxActivThisStop/calcPaxAlightS1 ==
  integrPax : Inport
  Subtract : Sum  Inputs=+-
  Unit Delay : UnitDelay  SampleTime=-1
  truPax : Outport
  intgPax : Outport  Port=2
  wires:
  integrPax/1 -> Unit Delay/1, intgPax/1, Subtract/1
  Subtract/1 -> truPax/1
  Unit Delay/1 -> Subtract/2

== system simRouteA_v4_11/atStopS14/calcPaxActivThisStop/calcPaxArrS1 ==
  integrPax : Inport
  Subtract : Sum  Inputs=+-
  Unit Delay : UnitDelay  SampleTime=-1
  truPax : Outport
  intgPax : Outport  Port=2
  wires:
  integrPax/1 -> Unit Delay/1, intgPax/1, Subtract/1
  Subtract/1 -> truPax/1
  Unit Delay/1 -> Subtract/2

== system simRouteA_v4_11/atStopS14/integrPaxAlightS1/Atomic Subsystem1 ==
  In1 : Inport
  Add : Sum
  Unit Delay : UnitDelay  SampleTime=-1
  Out1 : Outport
  wires:
  In1/1 -> Add/1
  Add/1 -> Out1/1, Unit Delay/1
  Unit Delay/1 -> Add/2

== system simRouteA_v4_11/atStopS14/integrPaxArrS1/Atomic Subsystem1 ==
  In1 : Inport
  Add : Sum
  Unit Delay : UnitDelay  SampleTime=-1
  Out1 : Outport
  wires:
  In1/1 -> Add/1
  Add/1 -> Out1/1, Unit Delay/1
  Unit Delay/1 -> Add/2

== system simRouteA_v4_11/atStopS15/busDwellThisStop/Subsystem2 ==
  dwellTime : Inport
  tStartSrvPax : Inport  Port=2
  Add1 : Sum
  Add2 : Sum
  Subtract : Sum  Inputs=+-
  Subtract1 : Sum  Inputs=+-
  Switch : Switch  Criteria=u2 > Threshold
  Unit Delay : UnitDelay  SampleTime=-1
  headWay : Constant  Value=3
  dwellTimeNew : Outport
  wires:
  Subtract/1 -> Switch/2
  Switch/1 -> Subtract1/1, Unit Delay/1
  headWay/1 -> Add2/1
  tStartSrvPax/1 -> Subtract1/2, Add1/2
  Add2/1 -> Switch/3
  dwellTime/1 -> Add1/1
  Subtract1/1 -> dwellTimeNew/1
  Add1/1 -> Switch/1, Subtract/1
  Unit Delay/1 -> Add2/2, Subtract/2

== system simRouteA_v4_11/atStopS15/calcPaxActivThisStop/Atomic Subsystem ==
  maxCap : Inport
  vacancy : Inport  Port=2
  paxAlight : Inport  Port=3
  paxArr : Inport  Port=4
  sec2Brd : Inport  Port=5
  Add : Sum
  Add1 : Sum
  Add2 : Sum
  Initial Value : InitialValue  Commented=on  InitialValue=0
  Min1 : MinMax  Inputs=2
  Min2 : MinMax  Inputs=2
  Product : Product
  Signal Latch : SignalLatch  Commented=on  MemoryWriteEdgeOption=Either  MemoryReadEdgeOption=Either  SpecifyReadEventPriority=on
      settings: InputPortMap=u0,u1,u2  OutputPortMap=o2
  Subtract : Sum  Inputs=+-
  Subtract1 : Sum  Inputs=-+
  Subtract2 : Sum  Inputs=+-
  Unit Delay : UnitDelay  SampleTime=-1
  newVacancy : Outport
  paxBoard : Outport  Port=2
  paxRemain : Outport  Port=3
  paxWait : Outport  Port=4
  dwellTime : Outport  Port=5
  corrPaxAlight : Outport  Port=6
  wires:
  Add/1 -> Min1/1, Subtract/1
  Min1/1 -> Subtract1/1, Subtract/2, Add2/1, paxBoard/1
  paxArr/1 -> Add1/1
  Add1/1 -> paxWait/1, Subtract1/2, Min1/2
  Subtract1/1 -> Unit Delay/1, paxRemain/1
  Unit Delay/1 -> Add1/2
  vacancy/1 -> Subtract2/2, Add/1
  maxCap/1 -> Subtract2/1
  Subtract/1 -> newVacancy/1
  Add2/1 -> Product/1
  sec2Brd/1 -> Product/2
  Product/1 -> dwellTime/1
  Subtract2/1 -> Min2/1
  Min2/1 -> corrPaxAlight/1, Add2/2, Add/2
  paxAlight/1 -> Min2/2

== system simRouteA_v4_11/atStopS15/calcPaxActivThisStop/calcPaxAlightS1 ==
  integrPax : Inport
  Subtract : Sum  Inputs=+-
  Unit Delay : UnitDelay  SampleTime=-1
  truPax : Outport
  intgPax : Outport  Port=2
  wires:
  integrPax/1 -> Unit Delay/1, intgPax/1, Subtract/1
  Subtract/1 -> truPax/1
  Unit Delay/1 -> Subtract/2

== system simRouteA_v4_11/atStopS15/calcPaxActivThisStop/calcPaxArrS1 ==
  integrPax : Inport
  Subtract : Sum  Inputs=+-
  Unit Delay : UnitDelay  SampleTime=-1
  truPax : Outport
  intgPax : Outport  Port=2
  wires:
  integrPax/1 -> Unit Delay/1, intgPax/1, Subtract/1
  Subtract/1 -> truPax/1
  Unit Delay/1 -> Subtract/2

== system simRouteA_v4_11/atStopS15/integrPaxAlightS1/Atomic Subsystem1 ==
  In1 : Inport
  Add : Sum
  Unit Delay : UnitDelay  SampleTime=-1
  Out1 : Outport
  wires:
  In1/1 -> Add/1
  Add/1 -> Out1/1, Unit Delay/1
  Unit Delay/1 -> Add/2

== system simRouteA_v4_11/atStopS15/integrPaxArrS1/Atomic Subsystem1 ==
  In1 : Inport
  Add : Sum
  Unit Delay : UnitDelay  SampleTime=-1
  Out1 : Outport
  wires:
  In1/1 -> Add/1
  Add/1 -> Out1/1, Unit Delay/1
  Unit Delay/1 -> Add/2

== system simRouteA_v4_11/atStopS16/busDwellThisStop/Subsystem2 ==
  dwellTime : Inport
  tStartSrvPax : Inport  Port=2
  Add1 : Sum
  Add2 : Sum
  Subtract : Sum  Inputs=+-
  Subtract1 : Sum  Inputs=+-
  Switch : Switch  Criteria=u2 > Threshold
  Unit Delay : UnitDelay  SampleTime=-1
  headWay : Constant  Value=3
  dwellTimeNew : Outport
  wires:
  Subtract/1 -> Switch/2
  Switch/1 -> Subtract1/1, Unit Delay/1
  headWay/1 -> Add2/1
  tStartSrvPax/1 -> Subtract1/2, Add1/2
  Add2/1 -> Switch/3
  dwellTime/1 -> Add1/1
  Subtract1/1 -> dwellTimeNew/1
  Add1/1 -> Switch/1, Subtract/1
  Unit Delay/1 -> Add2/2, Subtract/2

== system simRouteA_v4_11/atStopS16/calcPaxActivThisStop/Atomic Subsystem ==
  maxCap : Inport
  vacancy : Inport  Port=2
  paxAlight : Inport  Port=3
  paxArr : Inport  Port=4
  sec2Brd : Inport  Port=5
  Add : Sum
  Add1 : Sum
  Add2 : Sum
  Initial Value : InitialValue  Commented=on  InitialValue=0
  Min1 : MinMax  Inputs=2
  Min2 : MinMax  Inputs=2
  Product : Product
  Signal Latch : SignalLatch  Commented=on  MemoryWriteEdgeOption=Either  MemoryReadEdgeOption=Either  SpecifyReadEventPriority=on
      settings: InputPortMap=u0,u1,u2  OutputPortMap=o2
  Subtract : Sum  Inputs=+-
  Subtract1 : Sum  Inputs=-+
  Subtract2 : Sum  Inputs=+-
  Unit Delay : UnitDelay  SampleTime=-1
  newVacancy : Outport
  paxBoard : Outport  Port=2
  paxRemain : Outport  Port=3
  paxWait : Outport  Port=4
  dwellTime : Outport  Port=5
  corrPaxAlight : Outport  Port=6
  wires:
  Add/1 -> Min1/1, Subtract/1
  Min1/1 -> Subtract1/1, Subtract/2, Add2/1, paxBoard/1
  paxArr/1 -> Add1/1
  Add1/1 -> paxWait/1, Subtract1/2, Min1/2
  Subtract1/1 -> Unit Delay/1, paxRemain/1
  Unit Delay/1 -> Add1/2
  vacancy/1 -> Subtract2/2, Add/1
  maxCap/1 -> Subtract2/1
  Subtract/1 -> newVacancy/1
  Add2/1 -> Product/1
  sec2Brd/1 -> Product/2
  Product/1 -> dwellTime/1
  Subtract2/1 -> Min2/1
  Min2/1 -> corrPaxAlight/1, Add2/2, Add/2
  paxAlight/1 -> Min2/2

== system simRouteA_v4_11/atStopS16/calcPaxActivThisStop/calcPaxAlightS1 ==
  integrPax : Inport
  Subtract : Sum  Inputs=+-
  Unit Delay : UnitDelay  SampleTime=-1
  truPax : Outport
  intgPax : Outport  Port=2
  wires:
  integrPax/1 -> Unit Delay/1, intgPax/1, Subtract/1
  Subtract/1 -> truPax/1
  Unit Delay/1 -> Subtract/2

== system simRouteA_v4_11/atStopS16/calcPaxActivThisStop/calcPaxArrS1 ==
  integrPax : Inport
  Subtract : Sum  Inputs=+-
  Unit Delay : UnitDelay  SampleTime=-1
  truPax : Outport
  intgPax : Outport  Port=2
  wires:
  integrPax/1 -> Unit Delay/1, intgPax/1, Subtract/1
  Subtract/1 -> truPax/1
  Unit Delay/1 -> Subtract/2

== system simRouteA_v4_11/atStopS16/integrPaxAlightS1/Atomic Subsystem1 ==
  In1 : Inport
  Add : Sum
  Unit Delay : UnitDelay  SampleTime=-1
  Out1 : Outport
  wires:
  In1/1 -> Add/1
  Add/1 -> Out1/1, Unit Delay/1
  Unit Delay/1 -> Add/2

== system simRouteA_v4_11/atStopS16/integrPaxArrS1/Atomic Subsystem1 ==
  In1 : Inport
  Add : Sum
  Unit Delay : UnitDelay  SampleTime=-1
  Out1 : Outport
  wires:
  In1/1 -> Add/1
  Add/1 -> Out1/1, Unit Delay/1
  Unit Delay/1 -> Add/2

== system simRouteA_v4_11/atStopS17/busDwellThisStop/Subsystem2 ==
  dwellTime : Inport
  tStartSrvPax : Inport  Port=2
  Add1 : Sum
  Add2 : Sum
  Subtract : Sum  Inputs=+-
  Subtract1 : Sum  Inputs=+-
  Switch : Switch  Criteria=u2 > Threshold
  Unit Delay : UnitDelay  SampleTime=-1
  headWay : Constant  Value=3
  dwellTimeNew : Outport
  wires:
  Subtract/1 -> Switch/2
  Switch/1 -> Subtract1/1, Unit Delay/1
  headWay/1 -> Add2/1
  tStartSrvPax/1 -> Subtract1/2, Add1/2
  Add2/1 -> Switch/3
  dwellTime/1 -> Add1/1
  Subtract1/1 -> dwellTimeNew/1
  Add1/1 -> Switch/1, Subtract/1
  Unit Delay/1 -> Add2/2, Subtract/2

== system simRouteA_v4_11/atStopS17/calcPaxActivThisStop/Atomic Subsystem ==
  maxCap : Inport
  vacancy : Inport  Port=2
  paxAlight : Inport  Port=3
  paxArr : Inport  Port=4
  sec2Brd : Inport  Port=5
  Add : Sum
  Add1 : Sum
  Add2 : Sum
  Initial Value : InitialValue  Commented=on  InitialValue=0
  Min1 : MinMax  Inputs=2
  Min2 : MinMax  Inputs=2
  Product : Product
  Signal Latch : SignalLatch  Commented=on  MemoryWriteEdgeOption=Either  MemoryReadEdgeOption=Either  SpecifyReadEventPriority=on
      settings: InputPortMap=u0,u1,u2  OutputPortMap=o2
  Subtract : Sum  Inputs=+-
  Subtract1 : Sum  Inputs=-+
  Subtract2 : Sum  Inputs=+-
  Unit Delay : UnitDelay  SampleTime=-1
  newVacancy : Outport
  paxBoard : Outport  Port=2
  paxRemain : Outport  Port=3
  paxWait : Outport  Port=4
  dwellTime : Outport  Port=5
  corrPaxAlight : Outport  Port=6
  wires:
  Add/1 -> Min1/1, Subtract/1
  Min1/1 -> Subtract1/1, Subtract/2, Add2/1, paxBoard/1
  paxArr/1 -> Add1/1
  Add1/1 -> paxWait/1, Subtract1/2, Min1/2
  Subtract1/1 -> Unit Delay/1, paxRemain/1
  Unit Delay/1 -> Add1/2
  vacancy/1 -> Subtract2/2, Add/1
  maxCap/1 -> Subtract2/1
  Subtract/1 -> newVacancy/1
  Add2/1 -> Product/1
  sec2Brd/1 -> Product/2
  Product/1 -> dwellTime/1
  Subtract2/1 -> Min2/1
  Min2/1 -> corrPaxAlight/1, Add2/2, Add/2
  paxAlight/1 -> Min2/2

== system simRouteA_v4_11/atStopS17/calcPaxActivThisStop/calcPaxAlightS1 ==
  integrPax : Inport
  Subtract : Sum  Inputs=+-
  Unit Delay : UnitDelay  SampleTime=-1
  truPax : Outport
  intgPax : Outport  Port=2
  wires:
  integrPax/1 -> Unit Delay/1, intgPax/1, Subtract/1
  Subtract/1 -> truPax/1
  Unit Delay/1 -> Subtract/2

== system simRouteA_v4_11/atStopS17/calcPaxActivThisStop/calcPaxArrS1 ==
  integrPax : Inport
  Subtract : Sum  Inputs=+-
  Unit Delay : UnitDelay  SampleTime=-1
  truPax : Outport
  intgPax : Outport  Port=2
  wires:
  integrPax/1 -> Unit Delay/1, intgPax/1, Subtract/1
  Subtract/1 -> truPax/1
  Unit Delay/1 -> Subtract/2

== system simRouteA_v4_11/atStopS17/integrPaxAlightS1/Atomic Subsystem1 ==
  In1 : Inport
  Add : Sum
  Unit Delay : UnitDelay  SampleTime=-1
  Out1 : Outport
  wires:
  In1/1 -> Add/1
  Add/1 -> Out1/1, Unit Delay/1
  Unit Delay/1 -> Add/2

== system simRouteA_v4_11/atStopS17/integrPaxArrS1/Atomic Subsystem1 ==
  In1 : Inport
  Add : Sum
  Unit Delay : UnitDelay  SampleTime=-1
  Out1 : Outport
  wires:
  In1/1 -> Add/1
  Add/1 -> Out1/1, Unit Delay/1
  Unit Delay/1 -> Add/2

== system simRouteA_v4_11/atStopS18/busDwellThisStop/Subsystem2 ==
  dwellTime : Inport
  tStartSrvPax : Inport  Port=2
  Add1 : Sum
  Add2 : Sum
  Subtract : Sum  Inputs=+-
  Subtract1 : Sum  Inputs=+-
  Switch : Switch  Criteria=u2 > Threshold
  Unit Delay : UnitDelay  SampleTime=-1
  headWay : Constant  Value=3
  dwellTimeNew : Outport
  wires:
  Subtract/1 -> Switch/2
  Switch/1 -> Subtract1/1, Unit Delay/1
  headWay/1 -> Add2/1
  tStartSrvPax/1 -> Subtract1/2, Add1/2
  Add2/1 -> Switch/3
  dwellTime/1 -> Add1/1
  Subtract1/1 -> dwellTimeNew/1
  Add1/1 -> Switch/1, Subtract/1
  Unit Delay/1 -> Add2/2, Subtract/2
